simulink model "control_sim"  (R2017a)
settings: Solver=VariableStepAuto  StartTime=0.0  StopTime=10.0  RelTol=1e-3  EnableMultiTasking=on
values from neighbouring files (symbols this model uses):
  I_frame = 0.26*l^2    (= 0.00582624367936)    [main.m]
  I_wheel = 0.5*m_wheel*r_wheel^2    (= 0.00016224)    [main.m]
  K = lqr(linsys.A,linsys.B,Q,R)    [main.m]
  r_wheel = 104e-3    (= 0.104)    [main.m]
  z0 = [theta_rad_init; 0; 0; 0]    [main.m]
settings Model: Creator=pluspole  LastModifiedBy=pluspole
settings OptimizationCC: LifeSpan=inf
settings DebuggingCC: SFExecutionAtInitializationDiag=none

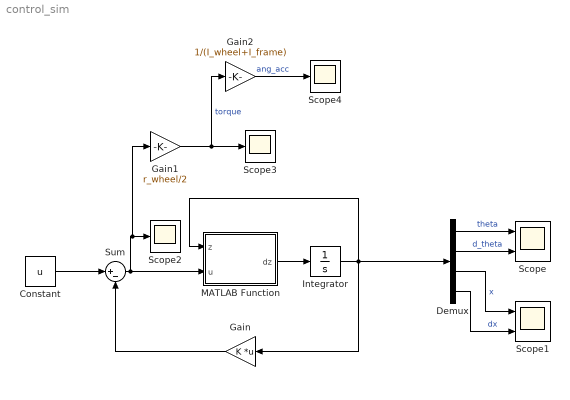
== system control_sim ==
  Constant : Constant  Value=u
  Demux : Demux
  Gain : Gain  Gain=K  Multiplication=Matrix(K*u) (u vector)
  Gain1 : Gain  Gain=r_wheel/2
  Gain2 : Gain  Gain=1/(I_wheel+I_frame)
  Integrator : Integrator  InitialCondition=z0
  MATLAB Function : MATLAB Function  TreatAsAtomicUnit=on
  Scope : Scope  NumInputPorts=2
  Scope1 : Scope  NumInputPorts=2
  Scope2 : Scope
  Scope3 : Scope
  Scope4 : Scope
  Sum : Sum  Inputs=|+-
  wires:
  MATLAB Function/1(dz) -> Integrator/1
  Sum/1 -> Gain1/1, Scope2/1, MATLAB Function/2(u)
  Gain/1 -> Sum/2
  Constant/1 -> Sum/1
  Integrator/1 -> Demux/1, Gain/1, MATLAB Function/1(z)
  Demux/1 -> Scope/1  "theta"
  Demux/2 -> Scope/2  "d_theta"
  Demux/3 -> Scope1/1  "x"
  Demux/4 -> Scope1/2  "dx"
  Gain1/1 -> Gain2/1, Scope3/1  "torque"
  Gain2/1 -> Scope4/1  "ang_acc"

== matlab function control_sim/MATLAB Function ==
  data: z input; u input; dz output; p parameter
function dz = fcn(z,u, p)

m=p.m;
M=p.M;
l=p.l;
g=p.g;
b=p.b;
k=p.k;

c1=cos(z(1));
s1=sin(z(1));

dz=zeros(4,1);

dz(1,1) = z(2);

dz(2,1) = ((u*c1)-(b*z(3)*c1)-((M+m)*g*s1)+(m*l*c1*s1*(z(2)^2))+((M+m)*((k*z(2))/(l*m))) )/(m*l*(c1^2)-((M+m)*l));
%dy(4,1) = (1/D)*((m+M)*m*g*L*Sy - m*L*Cy*(m*L*y(4)^2*Sy - d*y(2))) - m*L*Cy*(1/D)*u +.01*randn;

dz(3,1) = z(4);

dz(4,1) = (u-(b*z(3))+(m*l*s1*(z(2)^2))-(m*g*c1*s1)+(c1*(k/l)*z(2)))/((M+m)-(m*(c1^2)));
%dy(2,1) = (1/D)*(-m^2*L^2*g*Cy*Sy + m*L^2*(m*L*y(4)^2*Sy - d*y(2))) + m*L*L*(1/D)*u;
